simulink model "problem9"  (R2020a)
settings: Solver=VariableStepAuto  StartTime=0.0  StopTime=10.0  RelTol=1e-3
settings Model: Creator=Jake  LastModifiedBy=Jake

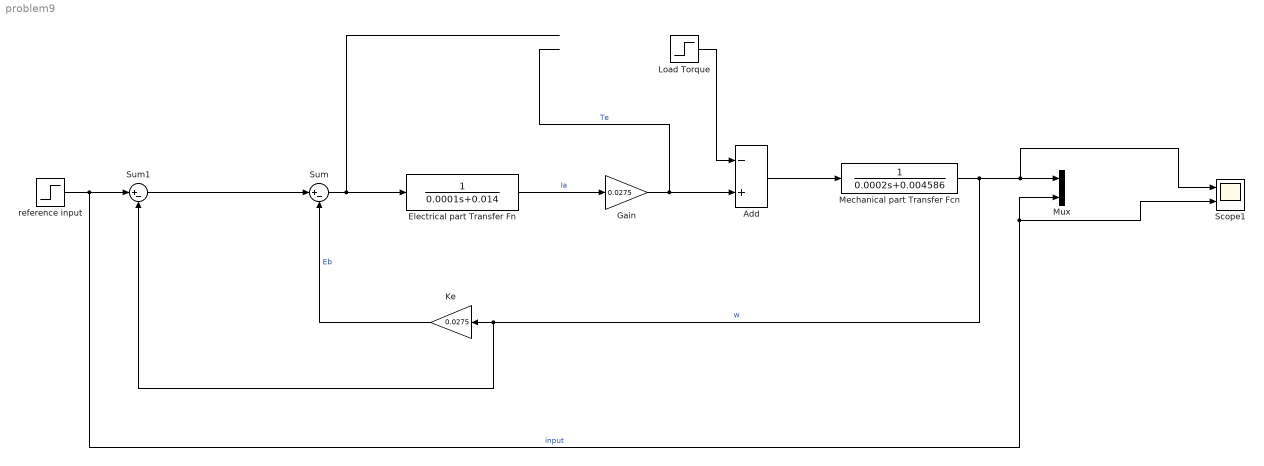
== system problem9 ==
  Add : Sum  Inputs=-+
  Electrical part Transfer Fn : TransferFcn  Denominator=[0.0001 0.014]
  Gain : Gain  Gain=0.0275
  Ke : Gain  Gain=0.0275
  Load Torque : Step  Time=0.1  After=10  SampleTime=0
  Mechanical part Transfer Fcn : TransferFcn  Denominator=[0.0002 0.004586]
  Mux : Mux  Inputs=2
  Scope1 : Scope  NumInputPorts=2
  Sum : Sum  Inputs=|+-
  Sum1 : Sum  Inputs=|+-
  reference input : Step  After=40  SampleTime=0
  wires:
  Gain/1 -> Add/2  "Te"
  Electrical part Transfer Fn/1 -> Gain/1  "Ia"
  Sum/1 -> Electrical part Transfer Fn/1
  Ke/1 -> Sum/2  "Eb"
  Add/1 -> Mechanical part Transfer Fcn/1
  Mechanical part Transfer Fcn/1 -> Scope1/1, Mux/1, Sum1/2, Ke/1  "w"
  Load Torque/1 -> Add/1
  reference input/1 -> Scope1/2, Mux/2, Sum1/1  "input"
  Sum1/1 -> Sum/1
